simulink model "A_Inverter_SVM_Simple_X_V3_OUR_Kit"  (Simulink 7.7)
settings: Solver=ode45  StartTime=0.0  StopTime=0.08  RelTol=1e-3
InitFcn:
  | clc;
  | 
  | f=50;           % Reference frequency
  | fs=4000;      % Switching frequency
  | m=1;           % Modulation index
libraries: xbsIndex_r4 x85, powerlib x13
Description:
  | This model simulates a simple space vector pulse width modulation technique
  | and plot space vector trajectory as well.
  | 
  | Syed Abdul Rahman Kashif
  | EED, UET, Lahore, Pakistan
settings Model: Creator=Abdul Rahman Kashif  LastModifiedBy=Administrator

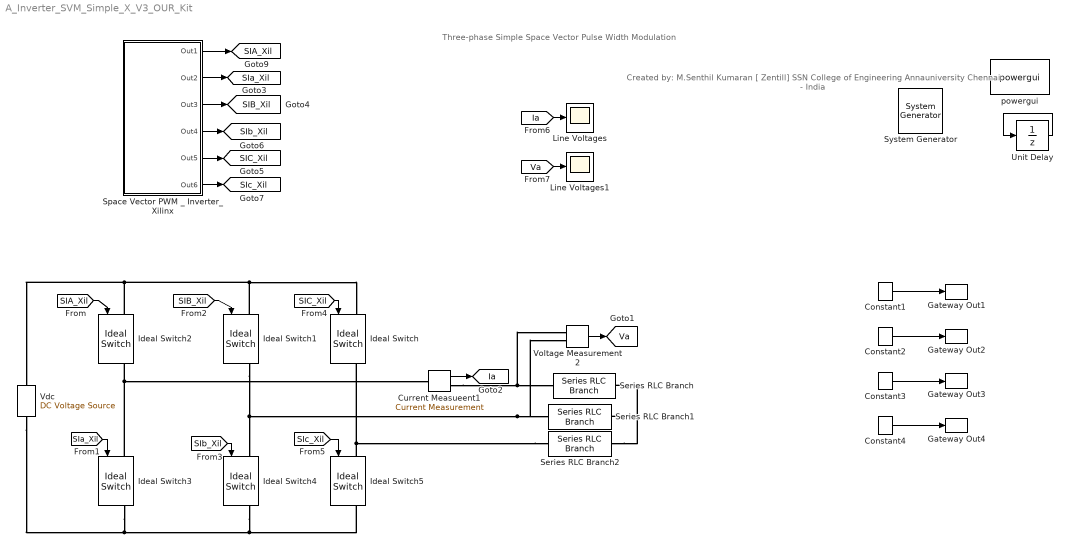
== system A_Inverter_SVM_Simple_X_V3_OUR_Kit ==
  note: Three-phase Simple Space Vector Pulse Width Modulation
  note: Created by: M.Senthil Kumaran [ Zentill]
      | SSN College of Engineering
      | Annauniversity
      | Chennai - India
  " System Generator" : xbsIndex_r4/ System Generator  Tag=genX  SystemSampleTime=-1  xilinxfamily=spartan3e  part=xc3s500e  speed=-4  package=fg320  synthesis_tool=XST  clock_wrapper=Clock Enables  directory=./vhdl  proj_type=Project Navigator  Synth_file=XST Defaults  Impl_file=ISE Defaults  testbench=off  simulink_period=20e-9  sysclk_period=20  dcm_input_clock_period=10  incr_netlist=off  trim_vbits=Everywhere in SubSystem  dbl_ovrd=According to Block Masks  core_generation=According to Block Masks  run_coregen=off  deprecated_control=off  eval_field=0  block_type=sysgen
  Constant1 : xbsIndex_r4/Constant  const=1  gui_display_data_type=Boolean  arith_type=Boolean  n_bits=1  bin_pt=0  preci_type=Single  exp_width=8  frac_width=24  explicit_period=on  period=120e-9  equ=P=C  opselect=C  inp2=PCIN>>17  opr=+  inp1=P  carry=CIN  dbl_ovrd=off  block_type=constant
  Constant2 : xbsIndex_r4/Constant  const=1  gui_display_data_type=Boolean  arith_type=Boolean  n_bits=1  bin_pt=0  preci_type=Single  exp_width=8  frac_width=24  explicit_period=on  period=120e-9  equ=P=C  opselect=C  inp2=PCIN>>17  opr=+  inp1=P  carry=CIN  dbl_ovrd=off  block_type=constant
  Constant3 : xbsIndex_r4/Constant  const=0  gui_display_data_type=Boolean  arith_type=Boolean  n_bits=1  bin_pt=0  preci_type=Single  exp_width=8  frac_width=24  explicit_period=on  period=120e-9  equ=P=C  opselect=C  inp2=PCIN>>17  opr=+  inp1=P  carry=CIN  dbl_ovrd=off  block_type=constant
  Constant4 : xbsIndex_r4/Constant  const=0  gui_display_data_type=Boolean  arith_type=Boolean  n_bits=1  bin_pt=0  preci_type=Single  exp_width=8  frac_width=24  explicit_period=on  period=120e-9  equ=P=C  opselect=C  inp2=PCIN>>17  opr=+  inp1=P  carry=CIN  dbl_ovrd=off  block_type=constant
  Current Measueent1 : powerlib/Measurements/Current Measurement  SystemSampleTime=-1  PhasorSimulation=off  OutputType=Complex  PSBequivalent=0
  Gateway Out1 : xbsIndex_r4/Gateway Out  inherit_from_input=off  hdl_port=on  timing_constraint=None  locs_specified=on  LOCs={'j14'}  UseAsDAC=off  DACChannel='1'  block_type=gatewayout
  Gateway Out2 : xbsIndex_r4/Gateway Out  inherit_from_input=off  hdl_port=on  timing_constraint=None  locs_specified=on  LOCs={'k14'}  UseAsDAC=off  DACChannel='1'  block_type=gatewayout
  Gateway Out3 : xbsIndex_r4/Gateway Out  inherit_from_input=off  hdl_port=on  timing_constraint=None  locs_specified=on  LOCs={'m15'}  UseAsDAC=off  DACChannel='1'  block_type=gatewayout
  Gateway Out4 : xbsIndex_r4/Gateway Out  inherit_from_input=off  hdl_port=on  timing_constraint=None  locs_specified=on  LOCs={'m16'}  UseAsDAC=off  DACChannel='1'  block_type=gatewayout
  Ideal Switch{,1..5} (6 alike) : powerlib/Power Electronics/Ideal Switch  SystemSampleTime=-1  Ron=0.001  Lon=0  IC=0  Rs=1e5  Cs=inf  Measurements=on
  Line Voltages : Scope
      settings: YMin=2.25  YMax=3.35  SaveName=Line_voltages  MaxDataPoints=5000000  SampleTime=2e-6
  Line Voltages1 : Scope
      settings: TimeRange=0.08  YMin=-400  YMax=25  SaveName=Line_voltages1  MaxDataPoints=5000000  SampleTime=2e-6
  Series RLC Branch : powerlib/Elements/Series RLC Branch  PhysicalDomain=powersysdomain  SubClassName=unknown  LeftPortType=p1  RightPortType=p1  LConnTagsString=__new0  RConnTagsString=__new0  BranchType=RL  Resistance=20  Inductance=27e-3  SetiL0=off  InitialCurrent=0  Capacitance=1e-6  Setx0=off  InitialVoltage=0  Measurements=None
  Series RLC Branch1 : powerlib/Elements/Series RLC Branch  PhysicalDomain=powersysdomain  SubClassName=unknown  LeftPortType=p1  RightPortType=p1  LConnTagsString=__new0  RConnTagsString=__new0  BranchType=RL  Resistance=20  Inductance=27e-3  SetiL0=off  InitialCurrent=0  Capacitance=1e-6  Setx0=off  InitialVoltage=0  Measurements=None
  Series RLC Branch2 : powerlib/Elements/Series RLC Branch  PhysicalDomain=powersysdomain  SubClassName=unknown  LeftPortType=p1  RightPortType=p1  LConnTagsString=__new0  RConnTagsString=__new0  BranchType=RL  Resistance=20  Inductance=27e-3  SetiL0=off  InitialCurrent=0  Capacitance=1e-6  Setx0=off  InitialVoltage=0  Measurements=None
  Space Vector PWM _ Inverter_ Xilinx : Subsystem
  Unit Delay : UnitDelay  SampleTime=1/4000000
  Vdc : powerlib/Electrical Sources/DC Voltage Source  SystemSampleTime=-1  Amplitude=400  Measurements=None
  Voltage Measurement2 : powerlib/Measurements/Voltage Measurement  SystemSampleTime=-1  PhasorSimulation=off  OutputType=Complex  PSBequivalent=0
  powergui : powerlib/powergui  Priority=1  SystemSampleTime=-1  SimulationMode=Continuous  SampleTime=50e-6  frequency=60  SPID=off  DisableSnubberDevices=off  DisableRonSwitches=off  DisableVfSwitches=off  SwTol=0  Interpol=off  DisplayEquations=off  FunctionMessages=off  frequencyindice=0  Pbase=100e6  ErrMax=1e-4  Iterations=50  UnitsV=kV  UnitsW=MW  echomessages=off  HookPort=off  EnableUseOfTLC=off  x0status=blocks  RestoreLinks=warning  ResistiveCurrentMeasurement=off  Ylog=off  Xlog=on  ShowGrid=off  save=off  variable=ZData  structure=Filtered_voltages  ZoomFFT=off  StartTime=0.02  cycles=1  DisplayStyle=1  fundamental=50  FreqAxis=off  MaxFrequency=1000  frequencyindicesteady=1  display=off  methode=off
  tag scope: Ia=global, SIA_Xil=global, SIB_Xil=global, SIC_Xil=global, SIa_Xil=global, SIb_Xil=global, SIc_Xil=global, Va=global
  wires:
  [SIA_Xil] -> Ideal Switch2/1
  [SIa_Xil] -> Ideal Switch3/1
  [SIB_Xil] -> Ideal Switch1/1
  [SIb_Xil] -> Ideal Switch4/1
  [SIC_Xil] -> Ideal Switch/1
  [SIc_Xil] -> Ideal Switch5/1
  Voltage Measurement2/1 -> [Va]
  Current Measueent1/1 -> [Ia]
  Unit Delay/1 -> Unit Delay/1
  [Ia] -> Line Voltages/1
  [Va] -> Line Voltages1/1
  Space Vector PWM _ Inverter_ Xilinx/1(Out1) -> [SIA_Xil]
  Space Vector PWM _ Inverter_ Xilinx/2(Out2) -> [SIa_Xil]
  Space Vector PWM _ Inverter_ Xilinx/3(Out3) -> [SIB_Xil]
  Space Vector PWM _ Inverter_ Xilinx/4(Out4) -> [SIb_Xil]
  Space Vector PWM _ Inverter_ Xilinx/5(Out5) -> [SIC_Xil]
  Space Vector PWM _ Inverter_ Xilinx/6(Out6) -> [SIc_Xil]
  Constant1/1 -> Gateway Out1/1
  Constant2/1 -> Gateway Out2/1
  Constant3/1 -> Gateway Out3/1
  Constant4/1 -> Gateway Out4/1
  connections:
  Ideal Switch3/LConn1 -- Ideal Switch2/RConn1 -- Current Measueent1/LConn1
  Series RLC Branch2/LConn1 -- Ideal Switch/RConn1 -- Ideal Switch5/LConn1
  Ideal Switch5/RConn1 -- Vdc/LConn1 -- Ideal Switch3/RConn1 -- Ideal Switch4/RConn1
  Ideal Switch1/RConn1 -- Ideal Switch4/LConn1 -- Series RLC Branch1/LConn1 -- Voltage Measurement2/LConn2
  Ideal Switch1/LConn1 -- Ideal Switch/LConn1 -- Ideal Switch2/LConn1 -- Vdc/RConn1
  Series RLC Branch/RConn1 -- Series RLC Branch1/RConn1 -- Series RLC Branch2/RConn1
  Current Measueent1/RConn1 -- Series RLC Branch/LConn1 -- Voltage Measurement2/LConn1

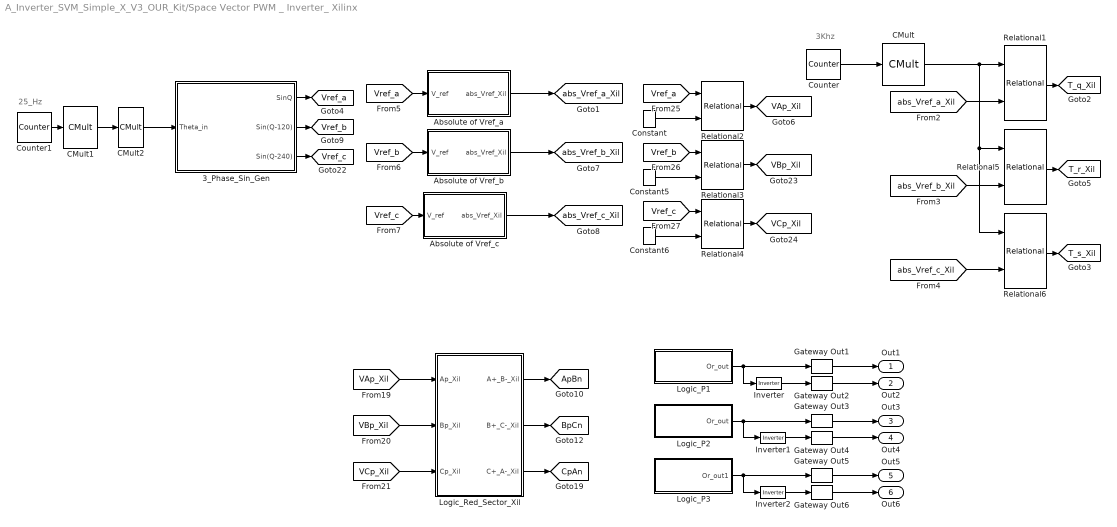
== system A_Inverter_SVM_Simple_X_V3_OUR_Kit/Space Vector PWM _ Inverter_ Xilinx ==
  note: 3Khz
  note: 25_Hz
  3_Phase_Sin_Gen : Subsystem
  Absolute of Vref_a : Subsystem
  Absolute of Vref_b : Subsystem
  Absolute of Vref_c : Subsystem
  CMult : xbsIndex_r4/CMult  const=5.99e-5  gui_display_data_type=Fixed-point  const_n_bits=24  const_bin_pt=24  float_type=Single  exp_bits=8  fraction_bits=24  en=off  latency=0  precision=User Defined  arith_type="Signed  (2's comp)"  n_bits=15  bin_pt=14  quantization=Truncate  overflow=Wrap  dbl_ovrd=off  use_behavioral_HDL=off  mem_type=Distributed RAM  pipeline=off  block_type=cmult
  CMult1 : xbsIndex_r4/CMult  const=1.499e-6  gui_display_data_type=Fixed-point  const_n_bits=29  const_bin_pt=29  float_type=Single  exp_bits=8  fraction_bits=24  en=off  latency=0  precision=User Defined  arith_type="Signed  (2's comp)"  n_bits=15  bin_pt=14  quantization=Truncate  overflow=Wrap  dbl_ovrd=off  use_behavioral_HDL=off  mem_type=Distributed RAM  pipeline=off  block_type=cmult
  CMult2 : xbsIndex_r4/CMult  const=360  gui_display_data_type=Fixed-point  const_n_bits=9  const_bin_pt=0  float_type=Single  exp_bits=8  fraction_bits=24  en=off  latency=0  precision=User Defined  arith_type=Unsigned  n_bits=9  bin_pt=0  quantization=Truncate  overflow=Wrap  dbl_ovrd=off  use_behavioral_HDL=off  mem_type=Distributed RAM  pipeline=off  block_type=cmult
  Constant : xbsIndex_r4/Constant  const=0  gui_display_data_type=Fixed-point  arith_type=Unsigned  n_bits=1  bin_pt=0  preci_type=Single  exp_width=8  frac_width=24  explicit_period=on  period=60e-9  equ=P=C  opselect=C  inp2=PCIN>>17  opr=+  inp1=P  carry=CIN  dbl_ovrd=off  block_type=constant
  Constant5 : xbsIndex_r4/Constant  const=0  gui_display_data_type=Fixed-point  arith_type=Unsigned  n_bits=1  bin_pt=0  preci_type=Single  exp_width=8  frac_width=24  explicit_period=on  period=60e-9  equ=P=C  opselect=C  inp2=PCIN>>17  opr=+  inp1=P  carry=CIN  dbl_ovrd=off  block_type=constant
  Constant6 : xbsIndex_r4/Constant  const=0  gui_display_data_type=Fixed-point  arith_type=Unsigned  n_bits=1  bin_pt=0  preci_type=Single  exp_width=8  frac_width=24  explicit_period=on  period=60e-9  equ=P=C  opselect=C  inp2=PCIN>>17  opr=+  inp1=P  carry=CIN  dbl_ovrd=off  block_type=constant
  Counter : xbsIndex_r4/Counter  cnt_type=Count Limited  cnt_to=16667  operation=Up  start_count=0  cnt_by_val=1  arith_type=Unsigned  n_bits=15  bin_pt=0  load_pin=off  rst=off  en=off  explicit_period=on  period=20e-9  dbl_ovrd=off  use_behavioral_HDL=off  implementation=Fabric  block_type=counter
  Counter1 : xbsIndex_r4/Counter  cnt_type=Count Limited  cnt_to=666667  operation=Up  start_count=0  cnt_by_val=1  arith_type=Unsigned  n_bits=20  bin_pt=0  load_pin=off  rst=off  en=off  explicit_period=on  period=60e-9  dbl_ovrd=off  use_behavioral_HDL=off  implementation=Fabric  block_type=counter
  Gateway Out1 : xbsIndex_r4/Gateway Out  inherit_from_input=off  hdl_port=on  timing_constraint=None  locs_specified=on  LOCs={'L15'}  UseAsDAC=off  DACChannel='1'  block_type=gatewayout
  Gateway Out2 : xbsIndex_r4/Gateway Out  inherit_from_input=off  hdl_port=on  timing_constraint=None  locs_specified=on  LOCs={'k13'}  UseAsDAC=off  DACChannel='1'  block_type=gatewayout
  Gateway Out3 : xbsIndex_r4/Gateway Out  inherit_from_input=off  hdl_port=on  timing_constraint=None  locs_specified=on  LOCs={'k12'}  UseAsDAC=off  DACChannel='1'  block_type=gatewayout
  Gateway Out4 : xbsIndex_r4/Gateway Out  inherit_from_input=off  hdl_port=on  timing_constraint=None  locs_specified=on  LOCs={'l16'}  UseAsDAC=off  DACChannel='1'  block_type=gatewayout
  Gateway Out5 : xbsIndex_r4/Gateway Out  inherit_from_input=off  hdl_port=on  timing_constraint=None  locs_specified=on  LOCs={'l17'}  UseAsDAC=off  DACChannel='1'  block_type=gatewayout
  Gateway Out6 : xbsIndex_r4/Gateway Out  inherit_from_input=off  hdl_port=on  timing_constraint=None  locs_specified=on  LOCs={'m14'}  UseAsDAC=off  DACChannel='1'  block_type=gatewayout
  Inverter : xbsIndex_r4/Inverter  en=off  latency=0  dbl_ovrd=off  block_type=inv
  Inverter1 : xbsIndex_r4/Inverter  en=off  latency=0  dbl_ovrd=off  block_type=inv
  Inverter2 : xbsIndex_r4/Inverter  en=off  latency=0  dbl_ovrd=off  block_type=inv
  Logic_P1 : Subsystem
  Logic_P2 : Subsystem
  Logic_P3 : Subsystem
  Logic_Red_Sector_Xil : Subsystem
  Relational1 : xbsIndex_r4/Relational  mode=a>b  en=off  latency=0  dbl_ovrd=off  block_type=relational
  Relational2 : xbsIndex_r4/Relational  mode=a>=b  en=off  latency=0  dbl_ovrd=off  block_type=relational
  Relational3 : xbsIndex_r4/Relational  mode=a>=b  en=off  latency=0  dbl_ovrd=off  block_type=relational
  Relational4 : xbsIndex_r4/Relational  mode=a>=b  en=off  latency=0  dbl_ovrd=off  block_type=relational
  Relational5 : xbsIndex_r4/Relational  mode=a>b  en=off  latency=0  dbl_ovrd=off  block_type=relational
  Relational6 : xbsIndex_r4/Relational  mode=a>b  en=off  latency=0  dbl_ovrd=off  block_type=relational
  Out1 : Outport
  Out2 : Outport  Port=2
  Out3 : Outport  Port=3
  Out4 : Outport  Port=4
  Out5 : Outport  Port=5
  Out6 : Outport  Port=6
  tag scope: ApBn=global, BpCn=global, CpAn=global, T_q_Xil=global, T_r_Xil=global, T_s_Xil=global, VAp_Xil=global, VBp_Xil=global, VCp_Xil=global, Vref_a=global, Vref_b=global, Vref_c=global, abs_Vref_a_Xil=global, abs_Vref_b_Xil=global, abs_Vref_c_Xil=global
  wires:
  Absolute of Vref_a/1(abs_Vref_Xil) -> [abs_Vref_a_Xil]
  Relational1/1 -> [T_q_Xil]
  Relational5/1 -> [T_r_Xil]
  Relational6/1 -> [T_s_Xil]
  [abs_Vref_a_Xil] -> Relational1/2
  Constant/1 -> Relational2/2
  Relational2/1 -> [VAp_Xil]
  [VAp_Xil] -> Logic_Red_Sector_Xil/1(Ap_Xil)
  [VBp_Xil] -> Logic_Red_Sector_Xil/2(Bp_Xil)
  [VCp_Xil] -> Logic_Red_Sector_Xil/3(Cp_Xil)
  Logic_Red_Sector_Xil/2(B+_C-_Xil) -> [BpCn]
  Logic_Red_Sector_Xil/3(C+_A-_Xil) -> [CpAn]
  Logic_P1/1(Or_out) -> Inverter/1, Gateway Out1/1
  Inverter/1 -> Gateway Out2/1
  Logic_P2/1(Or_out) -> Inverter1/1, Gateway Out3/1
  Inverter1/1 -> Gateway Out4/1
  Logic_P3/1(Or_out1) -> Inverter2/1, Gateway Out5/1
  Inverter2/1 -> Gateway Out6/1
  Logic_Red_Sector_Xil/1(A+_B-_Xil) -> [ApBn]
  Counter/1 -> CMult/1
  CMult/1 -> Relational1/1, Relational5/1, Relational6/1
  [Vref_a] -> Relational2/1
  Constant5/1 -> Relational3/2
  Relational3/1 -> [VBp_Xil]
  [Vref_b] -> Relational3/1
  Constant6/1 -> Relational4/2
  Relational4/1 -> [VCp_Xil]
  [Vref_c] -> Relational4/1
  [abs_Vref_b_Xil] -> Relational5/2
  [abs_Vref_c_Xil] -> Relational6/2
  [Vref_a] -> Absolute of Vref_a/1(V_ref)
  Absolute of Vref_b/1(abs_Vref_Xil) -> [abs_Vref_b_Xil]
  [Vref_b] -> Absolute of Vref_b/1(V_ref)
  Absolute of Vref_c/1(abs_Vref_Xil) -> [abs_Vref_c_Xil]
  [Vref_c] -> Absolute of Vref_c/1(V_ref)
  Gateway Out1/1 -> Out1/1
  Gateway Out2/1 -> Out2/1
  Gateway Out3/1 -> Out3/1
  Gateway Out4/1 -> Out4/1
  Gateway Out5/1 -> Out5/1
  Gateway Out6/1 -> Out6/1
  Counter1/1 -> CMult1/1
  CMult1/1 -> CMult2/1
  CMult2/1 -> 3_Phase_Sin_Gen/1(Theta_in)
  3_Phase_Sin_Gen/1(SinQ) -> [Vref_a]
  3_Phase_Sin_Gen/2(Sin(Q-120)) -> [Vref_b]
  3_Phase_Sin_Gen/3(Sin(Q-240)) -> [Vref_c]

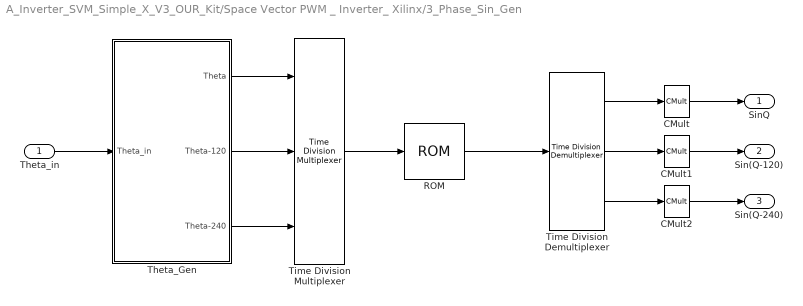
== system A_Inverter_SVM_Simple_X_V3_OUR_Kit/Space Vector PWM _ Inverter_ Xilinx/3_Phase_Sin_Gen ==
  Theta_in : Inport
  CMult : xbsIndex_r4/CMult  const=0.5  gui_display_data_type=Fixed-point  const_n_bits=2  const_bin_pt=2  float_type=Single  exp_bits=8  fraction_bits=24  en=off  latency=0  precision=Full  arith_type="Signed  (2's comp)"  n_bits=16  bin_pt=14  quantization=Truncate  overflow=Wrap  dbl_ovrd=off  use_behavioral_HDL=off  mem_type=Distributed RAM  pipeline=off  block_type=cmult
  CMult1 : xbsIndex_r4/CMult  const=0.5  gui_display_data_type=Fixed-point  const_n_bits=2  const_bin_pt=2  float_type=Single  exp_bits=8  fraction_bits=24  en=off  latency=0  precision=Full  arith_type="Signed  (2's comp)"  n_bits=16  bin_pt=14  quantization=Truncate  overflow=Wrap  dbl_ovrd=off  use_behavioral_HDL=off  mem_type=Distributed RAM  pipeline=off  block_type=cmult
  CMult2 : xbsIndex_r4/CMult  const=0.5  gui_display_data_type=Fixed-point  const_n_bits=2  const_bin_pt=2  float_type=Single  exp_bits=8  fraction_bits=24  en=off  latency=0  precision=Full  arith_type="Signed  (2's comp)"  n_bits=16  bin_pt=14  quantization=Truncate  overflow=Wrap  dbl_ovrd=off  use_behavioral_HDL=off  mem_type=Distributed RAM  pipeline=off  block_type=cmult
  ROM : xbsIndex_r4/ROM  depth=361  initVector=sin(2*pi*(0:360)/360)  distributed_mem=Distributed memory  rst=off  init_reg=0  en=off  latency=0  gui_display_data_type=Fixed-point  arith_type="Signed  (2's comp)"  n_bits=15  bin_pt=10  preci_type=Single  exp_width=8  frac_width=24  dbl_ovrd=off  optimize=Area  use_rpm=on  block_type=sprom
      settings: xl_use_area=on
  Theta_Gen : Subsystem
  Time Division Demultiplexer : xbsIndex_r4/Time Division Demultiplexer  frame_pattern=[1 1 1]  impl_style=Multiple Channel  vin=off  dbl_ovrd=off  explicit_period=off  period=1  block_type=tdd
      settings: infoedit=Samples presented at the input are selected and down-sampled according to the frame sampling pattern specified. The sampled input is presented either as a single or multiple channel at the output.
  Time Division Multiplexer : xbsIndex_r4/Time Division Multiplexer  inputs=3  vin=off  dbl_ovrd=off  explicit_period=off  period=1  block_type=tdm
      settings: infoedit="Multiple inputs are sampled and  presented serially at the output."
  SinQ : Outport
  Sin(Q-120) : Outport  Port=2
  Sin(Q-240) : Outport  Port=3
  wires:
  Theta_in/1 -> Theta_Gen/1(Theta_in)
  Theta_Gen/3(Theta-240) -> Time Division Multiplexer/3
  Theta_Gen/2(Theta-120) -> Time Division Multiplexer/2
  Theta_Gen/1(Theta) -> Time Division Multiplexer/1
  Time Division Demultiplexer/2 -> CMult1/1
  Time Division Multiplexer/1 -> ROM/1
  ROM/1 -> Time Division Demultiplexer/1
  Time Division Demultiplexer/3 -> CMult2/1
  Time Division Demultiplexer/1 -> CMult/1
  CMult/1 -> SinQ/1
  CMult1/1 -> Sin(Q-120)/1
  CMult2/1 -> Sin(Q-240)/1

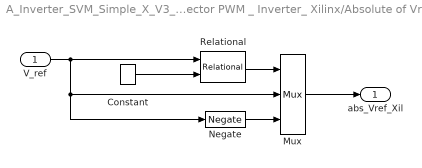
== system A_Inverter_SVM_Simple_X_V3_OUR_Kit/Space Vector PWM _ Inverter_ Xilinx/Absolute of Vref_a ==
  V_ref : Inport
  Constant : xbsIndex_r4/Constant  const=0  gui_display_data_type=Fixed-point  arith_type=Unsigned  n_bits=1  bin_pt=0  preci_type=Single  exp_width=8  frac_width=24  explicit_period=on  period=60e-9  equ=P=C  opselect=C  inp2=PCIN>>17  opr=+  inp1=P  carry=CIN  dbl_ovrd=off  block_type=constant
  Mux : xbsIndex_r4/Mux  inputs=2  en=off  latency=0  precision=User Defined  arith_type=Unsigned  n_bits=15  bin_pt=10  quantization=Truncate  overflow=Wrap  dbl_ovrd=off  block_type=mux
  Negate : xbsIndex_r4/Negate  precision=User Defined  arith_type=Unsigned  n_bits=15  bin_pt=10  quantization=Truncate  overflow=Wrap  en=off  latency=0  dbl_ovrd=off  block_type=negate
  Relational : xbsIndex_r4/Relational  mode=a<b  en=off  latency=0  dbl_ovrd=off  block_type=relational
  abs_Vref_Xil : Outport
  wires:
  Constant/1 -> Relational/2
  Relational/1 -> Mux/1
  Negate/1 -> Mux/3
  V_ref/1 -> Mux/2, Negate/1, Relational/1
  Mux/1 -> abs_Vref_Xil/1

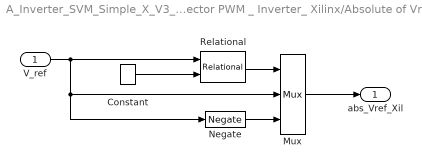
== system A_Inverter_SVM_Simple_X_V3_OUR_Kit/Space Vector PWM _ Inverter_ Xilinx/Absolute of Vref_b ==
  V_ref : Inport
  Constant : xbsIndex_r4/Constant  const=0  gui_display_data_type=Fixed-point  arith_type=Unsigned  n_bits=1  bin_pt=0  preci_type=Single  exp_width=8  frac_width=24  explicit_period=on  period=60e-9  equ=P=C  opselect=C  inp2=PCIN>>17  opr=+  inp1=P  carry=CIN  dbl_ovrd=off  block_type=constant
  Mux : xbsIndex_r4/Mux  inputs=2  en=off  latency=0  precision=User Defined  arith_type=Unsigned  n_bits=15  bin_pt=10  quantization=Truncate  overflow=Wrap  dbl_ovrd=off  block_type=mux
  Negate : xbsIndex_r4/Negate  precision=User Defined  arith_type=Unsigned  n_bits=15  bin_pt=10  quantization=Truncate  overflow=Wrap  en=off  latency=0  dbl_ovrd=off  block_type=negate
  Relational : xbsIndex_r4/Relational  mode=a<b  en=off  latency=0  dbl_ovrd=off  block_type=relational
  abs_Vref_Xil : Outport
  wires:
  Mux/1 -> abs_Vref_Xil/1
  V_ref/1 -> Relational/1, Negate/1, Mux/2
  Negate/1 -> Mux/3
  Relational/1 -> Mux/1
  Constant/1 -> Relational/2

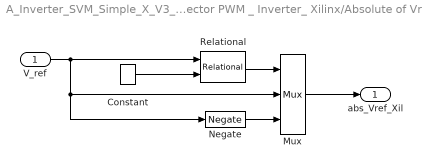
== system A_Inverter_SVM_Simple_X_V3_OUR_Kit/Space Vector PWM _ Inverter_ Xilinx/Absolute of Vref_c ==
  V_ref : Inport
  Constant : xbsIndex_r4/Constant  const=0  gui_display_data_type=Fixed-point  arith_type=Unsigned  n_bits=1  bin_pt=0  preci_type=Single  exp_width=8  frac_width=24  explicit_period=on  period=60e-9  equ=P=C  opselect=C  inp2=PCIN>>17  opr=+  inp1=P  carry=CIN  dbl_ovrd=off  block_type=constant
  Mux : xbsIndex_r4/Mux  inputs=2  en=off  latency=0  precision=User Defined  arith_type=Unsigned  n_bits=15  bin_pt=10  quantization=Truncate  overflow=Wrap  dbl_ovrd=off  block_type=mux
  Negate : xbsIndex_r4/Negate  precision=User Defined  arith_type=Unsigned  n_bits=15  bin_pt=10  quantization=Truncate  overflow=Wrap  en=off  latency=0  dbl_ovrd=off  block_type=negate
  Relational : xbsIndex_r4/Relational  mode=a<b  en=off  latency=0  dbl_ovrd=off  block_type=relational
  abs_Vref_Xil : Outport
  wires:
  Constant/1 -> Relational/2
  Relational/1 -> Mux/1
  Negate/1 -> Mux/3
  V_ref/1 -> Mux/2, Negate/1, Relational/1
  Mux/1 -> abs_Vref_Xil/1

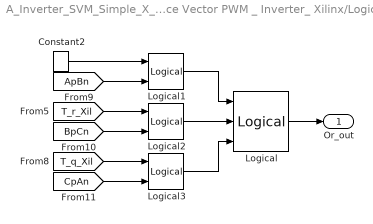
== system A_Inverter_SVM_Simple_X_V3_OUR_Kit/Space Vector PWM _ Inverter_ Xilinx/Logic_P1 ==
  Constant2 : xbsIndex_r4/Constant  const=1  gui_display_data_type=Boolean  arith_type=Boolean  n_bits=1  bin_pt=0  preci_type=Single  exp_width=8  frac_width=24  explicit_period=on  period=60e-9  equ=P=C  opselect=C  inp2=PCIN>>17  opr=+  inp1=P  carry=CIN  dbl_ovrd=off  block_type=constant
  Logical : xbsIndex_r4/Logical  logical_function=OR  inputs=3  en=off  latency=0  precision=Full  arith_type=Unsigned  n_bits=16  bin_pt=0  align_bp=on  dbl_ovrd=off  block_type=logical
  Logical1 : xbsIndex_r4/Logical  logical_function=AND  inputs=2  en=off  latency=0  precision=Full  arith_type=Unsigned  n_bits=16  bin_pt=0  align_bp=on  dbl_ovrd=off  block_type=logical
  Logical2 : xbsIndex_r4/Logical  logical_function=AND  inputs=2  en=off  latency=0  precision=Full  arith_type=Unsigned  n_bits=16  bin_pt=0  align_bp=on  dbl_ovrd=off  block_type=logical
  Logical3 : xbsIndex_r4/Logical  logical_function=AND  inputs=2  en=off  latency=0  precision=Full  arith_type=Unsigned  n_bits=16  bin_pt=0  align_bp=on  dbl_ovrd=off  block_type=logical
  Or_out : Outport
  wires:
  Logical2/1 -> Logical/2
  Logical3/1 -> Logical/3
  Logical1/1 -> Logical/1
  [ApBn] -> Logical1/2
  [T_r_Xil] -> Logical2/1
  Logical/1 -> Or_out/1
  [BpCn] -> Logical2/2
  [T_q_Xil] -> Logical3/1
  [CpAn] -> Logical3/2
  Constant2/1 -> Logical1/1

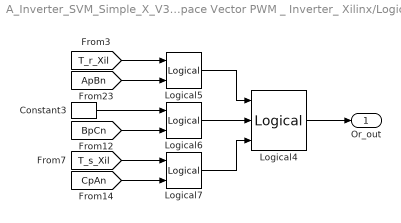
== system A_Inverter_SVM_Simple_X_V3_OUR_Kit/Space Vector PWM _ Inverter_ Xilinx/Logic_P2 ==
  Constant3 : xbsIndex_r4/Constant  const=1  gui_display_data_type=Boolean  arith_type=Boolean  n_bits=1  bin_pt=0  preci_type=Single  exp_width=8  frac_width=24  explicit_period=on  period=60e-9  equ=P=C  opselect=C  inp2=PCIN>>17  opr=+  inp1=P  carry=CIN  dbl_ovrd=off  block_type=constant
  Logical4 : xbsIndex_r4/Logical  logical_function=OR  inputs=3  en=off  latency=0  precision=Full  arith_type=Unsigned  n_bits=16  bin_pt=0  align_bp=on  dbl_ovrd=off  block_type=logical
  Logical5 : xbsIndex_r4/Logical  logical_function=AND  inputs=2  en=off  latency=0  precision=Full  arith_type=Unsigned  n_bits=16  bin_pt=0  align_bp=on  dbl_ovrd=off  block_type=logical
  Logical6 : xbsIndex_r4/Logical  logical_function=AND  inputs=2  en=off  latency=0  precision=Full  arith_type=Unsigned  n_bits=16  bin_pt=0  align_bp=on  dbl_ovrd=off  block_type=logical
  Logical7 : xbsIndex_r4/Logical  logical_function=AND  inputs=2  en=off  latency=0  precision=Full  arith_type=Unsigned  n_bits=16  bin_pt=0  align_bp=on  dbl_ovrd=off  block_type=logical
  Or_out : Outport
  wires:
  Logical6/1 -> Logical4/2
  Logical7/1 -> Logical4/3
  Logical5/1 -> Logical4/1
  [ApBn] -> Logical5/2
  Constant3/1 -> Logical6/1
  Logical4/1 -> Or_out/1
  [BpCn] -> Logical6/2
  [T_s_Xil] -> Logical7/1
  [CpAn] -> Logical7/2
  [T_r_Xil] -> Logical5/1

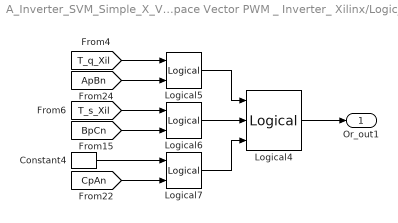
== system A_Inverter_SVM_Simple_X_V3_OUR_Kit/Space Vector PWM _ Inverter_ Xilinx/Logic_P3 ==
  Constant4 : xbsIndex_r4/Constant  const=1  gui_display_data_type=Boolean  arith_type=Boolean  n_bits=1  bin_pt=0  preci_type=Single  exp_width=8  frac_width=24  explicit_period=on  period=60e-9  equ=P=C  opselect=C  inp2=PCIN>>17  opr=+  inp1=P  carry=CIN  dbl_ovrd=off  block_type=constant
  Logical4 : xbsIndex_r4/Logical  logical_function=OR  inputs=3  en=off  latency=0  precision=Full  arith_type=Unsigned  n_bits=16  bin_pt=0  align_bp=on  dbl_ovrd=off  block_type=logical
  Logical5 : xbsIndex_r4/Logical  logical_function=AND  inputs=2  en=off  latency=0  precision=Full  arith_type=Unsigned  n_bits=16  bin_pt=0  align_bp=on  dbl_ovrd=off  block_type=logical
  Logical6 : xbsIndex_r4/Logical  logical_function=AND  inputs=2  en=off  latency=0  precision=Full  arith_type=Unsigned  n_bits=16  bin_pt=0  align_bp=on  dbl_ovrd=off  block_type=logical
  Logical7 : xbsIndex_r4/Logical  logical_function=AND  inputs=2  en=off  latency=0  precision=Full  arith_type=Unsigned  n_bits=16  bin_pt=0  align_bp=on  dbl_ovrd=off  block_type=logical
  Or_out1 : Outport
  wires:
  Logical6/1 -> Logical4/2
  Logical7/1 -> Logical4/3
  Logical5/1 -> Logical4/1
  [ApBn] -> Logical5/2
  [T_s_Xil] -> Logical6/1
  Logical4/1 -> Or_out1/1
  [BpCn] -> Logical6/2
  Constant4/1 -> Logical7/1
  [CpAn] -> Logical7/2
  [T_q_Xil] -> Logical5/1

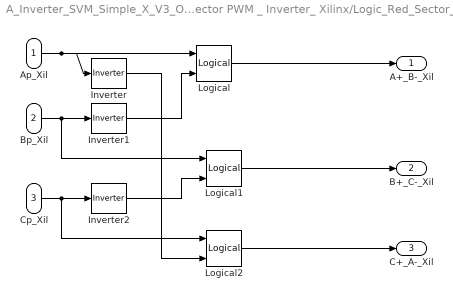
== system A_Inverter_SVM_Simple_X_V3_OUR_Kit/Space Vector PWM _ Inverter_ Xilinx/Logic_Red_Sector_Xil ==
  Ap_Xil : Inport
  Bp_Xil : Inport  Port=2
  Cp_Xil : Inport  Port=3
  Inverter : xbsIndex_r4/Inverter  en=off  latency=0  dbl_ovrd=off  block_type=inv
  Inverter1 : xbsIndex_r4/Inverter  en=off  latency=0  dbl_ovrd=off  block_type=inv
  Inverter2 : xbsIndex_r4/Inverter  en=off  latency=0  dbl_ovrd=off  block_type=inv
  Logical : xbsIndex_r4/Logical  logical_function=AND  inputs=2  en=off  latency=0  precision=Full  arith_type=Unsigned  n_bits=16  bin_pt=0  align_bp=on  dbl_ovrd=off  block_type=logical
  Logical1 : xbsIndex_r4/Logical  logical_function=AND  inputs=2  en=off  latency=0  precision=Full  arith_type=Unsigned  n_bits=16  bin_pt=0  align_bp=on  dbl_ovrd=off  block_type=logical
  Logical2 : xbsIndex_r4/Logical  logical_function=AND  inputs=2  en=off  latency=0  precision=Full  arith_type=Unsigned  n_bits=16  bin_pt=0  align_bp=on  dbl_ovrd=off  block_type=logical
  A+_B-_Xil : Outport
  B+_C-_Xil : Outport  Port=2
  C+_A-_Xil : Outport  Port=3
  wires:
  Ap_Xil/1 -> Inverter/1, Logical/1
  Inverter/1 -> Logical2/2
  Logical/1 -> A+_B-_Xil/1
  Logical1/1 -> B+_C-_Xil/1
  Bp_Xil/1 -> Inverter1/1, Logical1/1
  Logical2/1 -> C+_A-_Xil/1
  Cp_Xil/1 -> Inverter2/1, Logical2/1
  Inverter2/1 -> Logical1/2
  Inverter1/1 -> Logical/2

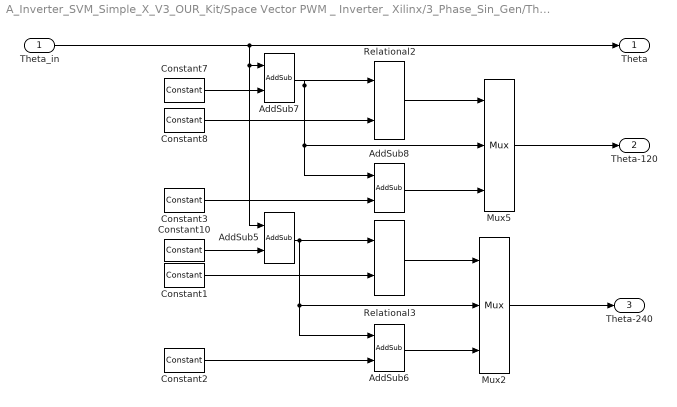
== system A_Inverter_SVM_Simple_X_V3_OUR_Kit/Space Vector PWM _ Inverter_ Xilinx/3_Phase_Sin_Gen/Theta_Gen ==
  Theta_in : Inport
  AddSub5 : xbsIndex_r4/AddSub  mode=Addition  use_carryin=off  use_carryout=off  en=off  latency=0  precision=User Defined  arith_type=Unsigned  n_bits=10  bin_pt=0  quantization=Truncate  overflow=Wrap  dbl_ovrd=off  use_behavioral_HDL=off  hw_selection=Fabric  pipelined=off  block_type=addsub
  AddSub6 : xbsIndex_r4/AddSub  mode=Subtraction  use_carryin=off  use_carryout=off  en=off  latency=0  precision=User Defined  arith_type=Unsigned  n_bits=8  bin_pt=0  quantization=Truncate  overflow=Wrap  dbl_ovrd=off  use_behavioral_HDL=off  hw_selection=Fabric  pipelined=off  block_type=addsub
  AddSub7 : xbsIndex_r4/AddSub  mode=Addition  use_carryin=off  use_carryout=off  en=off  latency=0  precision=User Defined  arith_type=Unsigned  n_bits=9  bin_pt=0  quantization=Truncate  overflow=Wrap  dbl_ovrd=off  use_behavioral_HDL=off  hw_selection=Fabric  pipelined=off  block_type=addsub
  AddSub8 : xbsIndex_r4/AddSub  mode=Subtraction  use_carryin=off  use_carryout=off  en=off  latency=0  precision=Full  arith_type=Unsigned  n_bits=8  bin_pt=0  quantization=Truncate  overflow=Wrap  dbl_ovrd=off  use_behavioral_HDL=off  hw_selection=Fabric  pipelined=off  block_type=addsub
  Constant{1..3,8} (4 alike) : xbsIndex_r4/Constant  const=360  gui_display_data_type=Fixed-point  arith_type=Unsigned  n_bits=9  bin_pt=0  preci_type=Single  exp_width=8  frac_width=24  explicit_period=on  period=60e-9  equ=P=C  opselect=C  inp2=PCIN>>17  opr=+  inp1=P  carry=CIN  dbl_ovrd=off  block_type=constant
  Constant10 : xbsIndex_r4/Constant  const=240  gui_display_data_type=Fixed-point  arith_type=Unsigned  n_bits=8  bin_pt=0  preci_type=Single  exp_width=8  frac_width=24  explicit_period=on  period=60e-9  equ=P=C  opselect=C  inp2=PCIN>>17  opr=+  inp1=P  carry=CIN  dbl_ovrd=off  block_type=constant
  Constant7 : xbsIndex_r4/Constant  const=120  gui_display_data_type=Fixed-point  arith_type=Unsigned  n_bits=7  bin_pt=0  preci_type=Single  exp_width=8  frac_width=24  explicit_period=on  period=60e-9  equ=P=C  opselect=C  inp2=PCIN>>17  opr=+  inp1=P  carry=CIN  dbl_ovrd=off  block_type=constant
  Mux2 : xbsIndex_r4/Mux  inputs=2  en=off  latency=0  precision=User Defined  arith_type=Unsigned  n_bits=9  bin_pt=0  quantization=Truncate  overflow=Wrap  dbl_ovrd=off  block_type=mux
  Mux5 : xbsIndex_r4/Mux  inputs=2  en=off  latency=0  precision=User Defined  arith_type=Unsigned  n_bits=9  bin_pt=0  quantization=Truncate  overflow=Wrap  dbl_ovrd=off  block_type=mux
  Relational2 : xbsIndex_r4/Relational  mode=a>=b  en=off  latency=0  dbl_ovrd=off  block_type=relational
  Relational3 : xbsIndex_r4/Relational  mode=a>=b  en=off  latency=0  dbl_ovrd=off  block_type=relational
  Theta : Outport
  Theta-120 : Outport  Port=2
  Theta-240 : Outport  Port=3
  wires:
  Mux2/1 -> Theta-240/1
  Mux5/1 -> Theta-120/1
  Constant2/1 -> AddSub6/2
  AddSub6/1 -> Mux2/3
  Relational3/1 -> Mux2/1
  Constant1/1 -> Relational3/2
  AddSub5/1 -> Relational3/1, Mux2/2, AddSub6/1
  Constant10/1 -> AddSub5/2
  Constant3/1 -> AddSub8/2
  AddSub8/1 -> Mux5/3
  Relational2/1 -> Mux5/1
  Constant8/1 -> Relational2/2
  AddSub7/1 -> AddSub8/1, Mux5/2, Relational2/1
  Constant7/1 -> AddSub7/2
  Theta_in/1 -> Theta/1, AddSub5/1, AddSub7/1
